simulink model "new_algorithm_real2"  (R2023b)
settings: Solver=FixedStepAuto  StartTime=0.0  StopTime=inf  RelTol=1e-3  EnableMultiTasking=on
undefined symbols (not defined in the file): hw
libraries: raspberrypiAVlib x3, dspfdesign x2, matrix_library x2, dspadpt3 x1
settings Model: ExtModeTrigDuration=2  Creator=mykni  LastModifiedBy=mykni
settings SolverCC: PositivePriorityOrder=on
settings OptimizationCC: EnhancedBackFolding=on  PassReuseOutputArgsAs=Individual arguments  ZeroExternalMemoryAtStartup=off  ZeroInternalMemoryAtStartup=off  MaxStackSize=64  OptimizeBlockOrder=speed  DifferentSizesBufferReuse=on  OptimizationCustomize=off  EfficientTunableParamExpr=on
settings DebuggingCC: ParameterTunabilityLossMsg=error
settings HardwareCC: ProdBitPerPointer=32  ProdBitPerSizeT=32  ProdBitPerPtrDiffT=32  ProdLargestAtomicInteger=Long  ProdLargestAtomicFloat=Double  ProdWordSize=32  ProdLongLongMode=on  ProdHWDeviceType=ARM Compatible->ARM Cortex  UseEmbeddedCoderFeatures=off
settings RTWCC: Description=Embedded Coder  SystemTargetFile=ert.tlc  HardwareBoard=Raspberry Pi  TLCOptions="-aInlineSetEventsForThisBaseRateFcn=TLC_FALSE -aSuppressMultiTaskScheduler=TLC_FALSE  -aRateBasedStepFcn=0"  TemplateMakefile=ert_default_tmf  Toolchain=GNU GCC Embedded Linux  BuildConfiguration=Faster Runs
settings CodeAppCC: ForceParamTrailComments=on  IgnoreCustomStorageClasses=off  OperatorAnnotations=on  SimulinkDataObjDesc=on  SFDataObjDesc=on  MangleLength=10  InsertBlockDesc=on
settings ERTTargetCC: SupportNonInlinedSFcns=on  SupportVariableSizeSignals=on  ExtModeTransport=2  ExtModeStaticAlloc=on  ExtModeMexFile=ext_xcp  ExtModeIntrfLevel=Level2 - Open

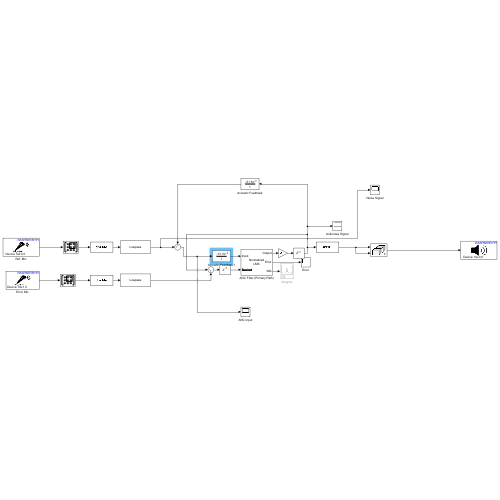
[thumbnail: Simulink's stored preview of the top-level diagram]
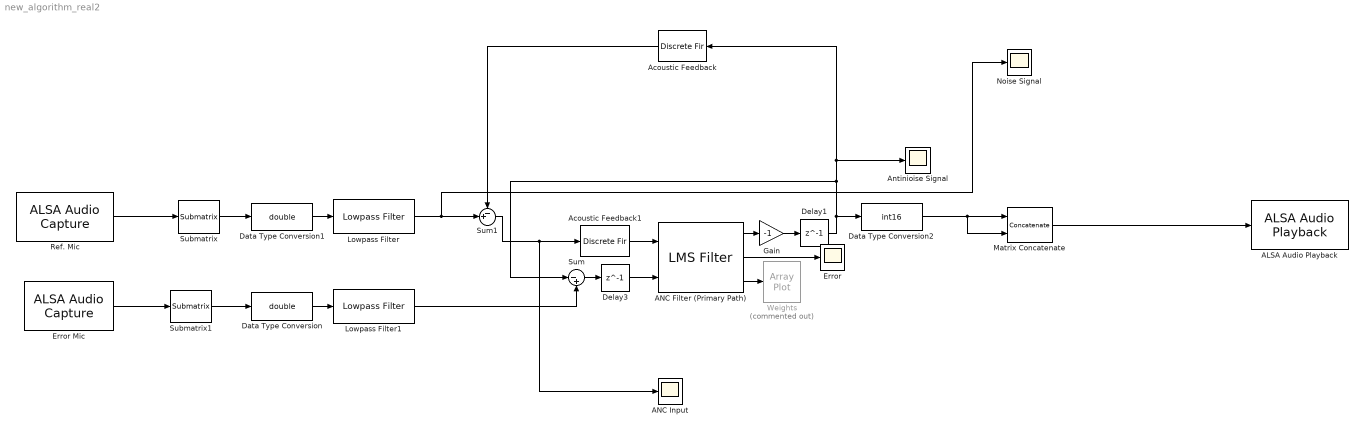
== system new_algorithm_real2 ==
  ALSA Audio Playback : raspberrypiAVlib/ALSA Audio Playback  deviceStr=hw:0,0  sampleRateEnum=44100  queueDuration=0.5  blockPlatform=LINUX
  ANC Filter (Primary Path) : dspadpt3/LMS Filter  Algo=Normalized LMS  L=32  stepflag=Dialog  mu=.005  leakage=1.0  ic=0  Adapt=off  resetflag=None  weights=on  addnparflag=off  roundingMode=Floor  overflowMode=off
  ANC Input : Scope
  Acoustic Feedback : DiscreteFir  Coefficients=[-.5 .5]  InputProcessing=Columns as channels (frame based)
  Acoustic Feedback1 : DiscreteFir  Coefficients=[-.5 .5]
  Antinioise Signal : Scope
  Data Type Conversion : DataTypeConversion  OutDataTypeStr=double  SaturateOnIntegerOverflow=off  RndMeth=Floor
  Data Type Conversion1 : DataTypeConversion  OutDataTypeStr=double  SaturateOnIntegerOverflow=off  RndMeth=Floor
  Data Type Conversion2 : DataTypeConversion  OutDataTypeStr=int16  SaturateOnIntegerOverflow=off  RndMeth=Floor
  Delay1 : Delay  DelayLength=1  InitialCondition=0
  Delay3 : Delay  DelayLength=1  InitialCondition=0
  Error : Scope
  Error Mic : raspberrypiAVlib/ALSA Audio Capture  deviceStr=hw:1,0  DataBitDepth=16-bit integer  numberOfChannels=2  sampleRateEnum=44100  frameSize=100  QueueDuration=0.5  blockPlatform=LINUX
  Gain : Gain  Gain=-1
  Lowpass Filter : dspfdesign/Lowpass Filter  FilterType=FIR  DesignForMinimumOrder=on  FilterOrder=50  PassbandFrequency=800  StopbandFrequency=1200  PassbandRipple=0.1  StopbandAttenuation=80  SampleRateMode=Specify on dialog  SampleRate=44100  SimulateUsing=Code generation  roundingMode=Floor  coeffsDataTypeStr=fixdt(1,16)
  Lowpass Filter1 : dspfdesign/Lowpass Filter  FilterType=FIR  DesignForMinimumOrder=on  FilterOrder=50  PassbandFrequency=800  StopbandFrequency=1200  PassbandRipple=0.1  StopbandAttenuation=80  SampleRateMode=Specify on dialog  SampleRate=44100  SimulateUsing=Code generation  roundingMode=Floor  coeffsDataTypeStr=fixdt(1,16)
  Matrix Concatenate : Concatenate  Mode=Multidimensional array  ConcatenateDimension=2
  Noise Signal : Scope
  Ref. Mic : raspberrypiAVlib/ALSA Audio Capture  deviceStr=hw:0,0  DataBitDepth=16-bit integer  numberOfChannels=2  sampleRateEnum=44100  frameSize=100  QueueDuration=0.5  blockPlatform=LINUX
  Submatrix : matrix_library/Submatrix  RowSpan=All rows  RowStartMode=First  RowStartIndex=1  RowEndMode=Last  RowEndIndex=1  ColSpan=One column  ColStartMode=First  ColStartIndex=1  ColEndMode=Last  ColEndIndex=1
  Submatrix1 : matrix_library/Submatrix  RowSpan=All rows  RowStartMode=First  RowStartIndex=1  RowEndMode=Last  RowEndIndex=1  ColSpan=One column  ColStartMode=First  ColStartIndex=1  ColEndMode=Last  ColEndIndex=1
  Sum : Sum  Inputs=|-+
  Sum1 : Sum  Inputs=-+|
  Weights : ArrayPlot  Commented=on  WindowPosition=[368.000000,182.000000,800.000000,500.000000,]  ScopeFrameLocation=window  YLimits=[-0.0551 0.1188]
  wires:
  Submatrix/1 -> Data Type Conversion1/1
  Matrix Concatenate/1 -> ALSA Audio Playback/1
  Submatrix1/1 -> Data Type Conversion/1
  Sum/1 -> Delay3/1
  Data Type Conversion2/1 -> Matrix Concatenate/2, Matrix Concatenate/1
  ANC Filter (Primary Path)/1 -> Gain/1
  Data Type Conversion1/1 -> Lowpass Filter/1
  Data Type Conversion/1 -> Lowpass Filter1/1
  Error Mic/1 -> Submatrix1/1
  ANC Filter (Primary Path)/3 -> Weights/1
  Ref. Mic/1 -> Submatrix/1
  ANC Filter (Primary Path)/2 -> Error/1
  Lowpass Filter1/1 -> Sum/2
  Gain/1 -> Delay1/1
  Delay1/1 -> Sum/1, Acoustic Feedback/1, Antinioise Signal/1, Data Type Conversion2/1
  Delay3/1 -> ANC Filter (Primary Path)/2
  Lowpass Filter/1 -> Sum1/2, Noise Signal/1
  Acoustic Feedback/1 -> Sum1/1
  Sum1/1 -> ANC Input/1, Acoustic Feedback1/1
  Acoustic Feedback1/1 -> ANC Filter (Primary Path)/1
